simulink model "cn0585_host_axi4_lite_read_write_example"  (R2021b)
settings: Solver=VariableStepAuto  StartTime=0.0  StopTime=10.0  RelTol=1e-3
undefined symbols (not defined in the file or in its folder): ip
libraries: axihostiiolib x4
settings Model: Creator=ppop  LastModifiedBy=ppop

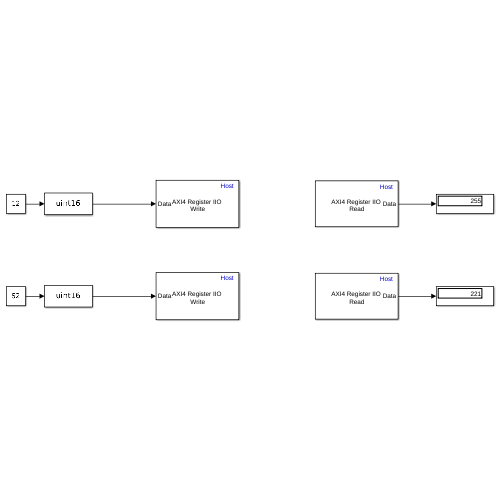
[thumbnail: Simulink's stored preview of the top-level diagram]
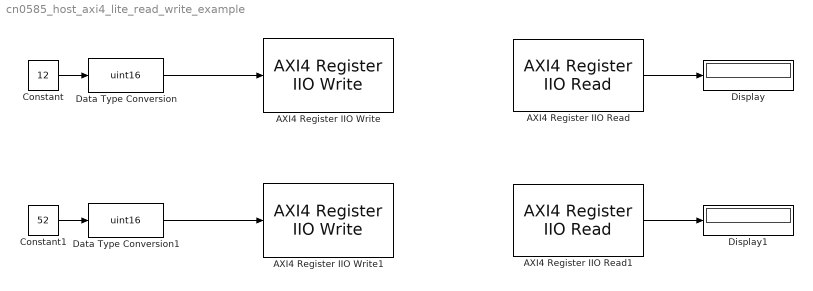
== system cn0585_host_axi4_lite_read_write_example ==
  AXI4 Register IIO Read : axihostiiolib/AXI4 Register IIO Read  devName=mwipcore0:mmrd-channel1  OutDataTypeStr=uint32  AddressOffset=hex2dec( '108' )  IPAddress=10.48.65.135  enIO=on  HardwareDataType=uint32  HardwareFixedPointDataTypeStr=fixdt(1,16,0)  uri=ip:10.48.65.135
      settings: SourceProductBaseCode=EMBEDDEDLINUX,INTEL_BLOCKSET,XILINX_BLOCKSET
  AXI4 Register IIO Read1 : axihostiiolib/AXI4 Register IIO Read  devName=mwipcore0:mmrd-channel1  OutDataTypeStr=uint32  AddressOffset=hex2dec( '10c' )  IPAddress=10.48.65.135  enIO=on  HardwareDataType=uint32  HardwareFixedPointDataTypeStr=fixdt(1,16,0)  uri=ip:10.48.65.135
      settings: SourceProductBaseCode=EMBEDDEDLINUX,INTEL_BLOCKSET,XILINX_BLOCKSET
  AXI4 Register IIO Write : axihostiiolib/AXI4 Register IIO Write  devName=mwipcore0:mmwr-channel0  AddressOffset=hex2dec( '100' )  IPAddress=10.48.65.135  uri=ip:10.48.65.135  enIO=on
      settings: SourceProductBaseCode=EMBEDDEDLINUX,INTEL_BLOCKSET,XILINX_BLOCKSET
  AXI4 Register IIO Write1 : axihostiiolib/AXI4 Register IIO Write  devName=mwipcore0:mmwr-channel0  AddressOffset=hex2dec( '104' )  IPAddress=10.48.65.135  uri=ip:10.48.65.135  enIO=on
      settings: SourceProductBaseCode=EMBEDDEDLINUX,INTEL_BLOCKSET,XILINX_BLOCKSET
  Constant : Constant  Value=12
  Constant1 : Constant  Value=52
  Data Type Conversion : DataTypeConversion  OutDataTypeStr=uint16
  Data Type Conversion1 : DataTypeConversion  OutDataTypeStr=uint16
  Display : Display
  Display1 : Display
  wires:
  AXI4 Register IIO Read/1 -> Display/1
  Data Type Conversion/1 -> AXI4 Register IIO Write/1
  Constant/1 -> Data Type Conversion/1
  Data Type Conversion1/1 -> AXI4 Register IIO Write1/1
  AXI4 Register IIO Read1/1 -> Display1/1
  Constant1/1 -> Data Type Conversion1/1
